simulink model "causalidad"  (R2023b)
settings: Solver=VariableStepAuto  StartTime=0.0  StopTime=10.0  RelTol=1e-3
settings Model: Creator=luisG  LastModifiedBy=diavl
settings OptimizationCC: ReuseModelBlockBuffer=off

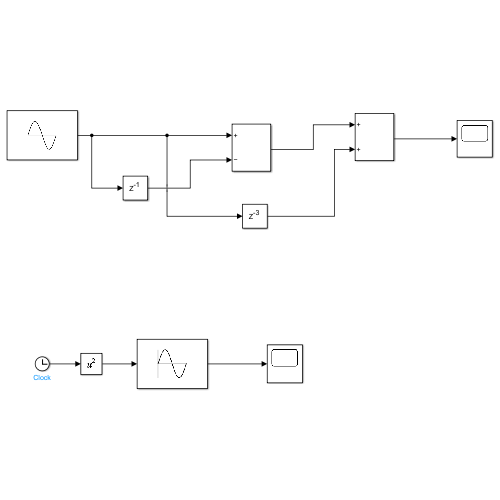
[thumbnail: Simulink's stored preview of the top-level diagram]
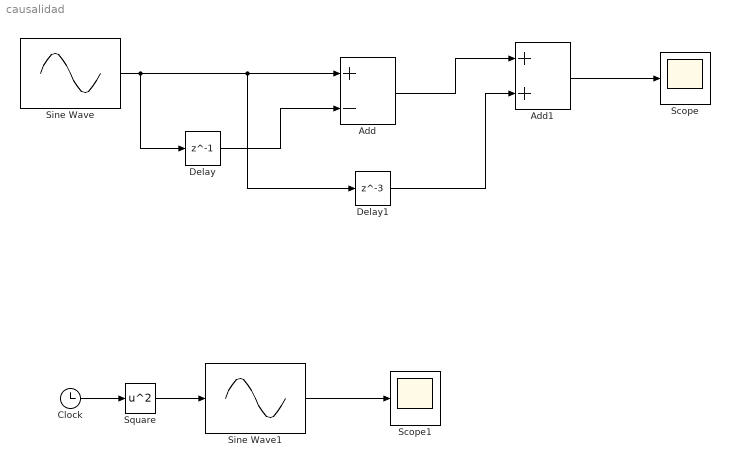
== system causalidad ==
  Add : Sum  Inputs=+-
  Add1 : Sum
  Clock : Clock
  Delay : Delay  DelayLength=1  InitialCondition=0
  Delay1 : Delay  DelayLength=3  InitialCondition=0
  Scope : Scope
  Scope1 : Scope
  Sine Wave : Sin  SampleTime=0
  Sine Wave1 : Sin  TimeSource=Use external signal  SampleTime=0
  Square : Math  Operator=square
  wires:
  Sine Wave/1 -> Delay/1, Delay1/1, Add/1
  Delay/1 -> Add/2
  Add/1 -> Add1/1
  Delay1/1 -> Add1/2
  Add1/1 -> Scope/1
  Square/1 -> Sine Wave1/1
  Clock/1 -> Square/1
  Sine Wave1/1 -> Scope1/1
